simulink model "Beleuchtungs_Box17b"  (R2017b)
settings: Solver=FixedStepAuto  StartTime=0.0  StopTime=10.0  RelTol=1e-3
PreLoadFcn:
  | waijung.modelPreload; % Required for working with Waijung Blockset. Do not remove.
undefined symbols (not defined in the file): HSEOSC, Link, LQFP176, ST, STM32F417IG
libraries: simulink x18, canmsglib x10, stm32f4_canbus_lib x2, stm32f4_io_lib x1, stm32f4_device_config_lib x1, hdlsllib x1
CloseFcn:
  | waijung.modelClose; % Required for working with Waijung Blockset. Do not remove.
settings Model: Creator=labadmin  LastModifiedBy=MichaelRogalski
settings OptimizationCC: DefaultParameterBehavior=Inlined  PassReuseOutputArgsAs=Individual arguments
settings DebuggingCC: ParameterTunabilityLossMsg=error
settings HardwareCC: ProdBitPerPointer=32  ProdBitPerSizeT=32  ProdBitPerPtrDiffT=32  ProdLargestAtomicFloat=None  ProdIntDivRoundTo=Undefined  ProdWordSize=32  ProdHWDeviceType=ARM Compatible->Cortex - M4  TargetEndianess=LittleEndian  TargetHWDeviceType=ARM Compatible->Cortex - M4
settings SFSimCC: MATLABDynamicMemAlloc=off
settings RTWCC: Description=STM32F4 Target  SystemTargetFile=stm32f4.tlc  GenerateMakefile=off  TemplateMakefile=ert_default_tmf  GenerateReport=on  IncludeHyperlinkInReport=on  LaunchReport=on  GenerateTraceInfo=on  GenerateTraceReport=on  GenerateTraceReportSl=on  GenerateTraceReportSf=on  GenerateTraceReportEml=on
settings CodeAppCC: ForceParamTrailComments=on  IgnoreCustomStorageClasses=off  OperatorAnnotations=on  SimulinkDataObjDesc=on  SFDataObjDesc=on  InsertBlockDesc=on
settings STFCustomTargetCC: TargetLangStandard=C99 (ISO)  MultiwordLength=256  ModelReferenceCompliant=off  CombineOutputUpdateFcns=on  ERTCustomFileBanners=on  SupportContinuousTime=off  SupportNonInlinedSFcns=off  RemoveResetFunc=on  MATLABClassNameForMDSCustomization=Simulink.SoftwareTarget.ERTCustomization  GRTInterface=off  SystemTargetFile=stm32f4.tlc
settings ERTTargetCC: TargetLangStandard=C99 (ISO)  ModelReferenceCompliant=off  ParMdlRefBuildCompliant=off  CompOptLevelCompliant=off  ConcurrentExecutionCompliant=off  ModelStepFunctionPrototypeControlCompliant=off  CPPClassGenCompliant=off  UseToolchainInfoCompliant=off  InlinedParameterPlacement=NonHierarchical  ERTSrcFileBannerTemplate=stm32f4_code_template.cgt  ERTHdrFileBannerTemplate=stm32f4_code_template.cgt  ERTDataSrcFileTemplate=stm32f4_code_template.cgt  ERTDataHdrFileTemplate=stm32f4_code_template.cgt  ERTCustomFileTemplate=stm32f4_file_process.tlc

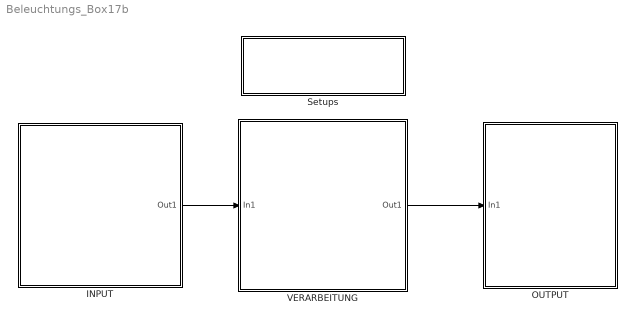
== system Beleuchtungs_Box17b ==
  INPUT : Subsystem
  OUTPUT : Subsystem
  Setups : Subsystem
  VERARBEITUNG : Subsystem
  wires:
  INPUT/1(Out1) -> VERARBEITUNG/1(In1)
  VERARBEITUNG/1(Out1) -> OUTPUT/1(In1)

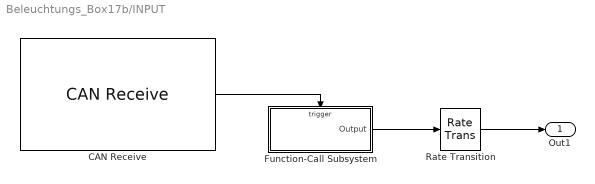
== system Beleuchtungs_Box17b/INPUT ==
  CAN Receive : stm32f4_canbus_lib/CAN Receive  conf=Rx  canmodule=1  idtype=Standard  filtertype=Mask  id=0  idmask=0  enableisr=on  usedlc=off  datatype=single  data0type=uint32  data1type=uint32  data2type=Not used  data3type=Not used  data4type=Not used  data5type=Not used  data6type=Not used  data7type=Not used  buffersize=8  sampletime=-1  sampletimestr=-1  blockid=INPUTCANReceive  inputarray=[]  inputlabelarray={}  outputarray=[7]  outputlabelarray={'Call ISR' }  compat=0  confstr=[]
      settings: SourceProductName=Waijung Blockset
  Function-Call Subsystem : Subsystem  TreatAsAtomicUnit=on
  Rate Transition : RateTransition
  Out1 : Outport  VectorParamsAs1DForOutWhenUnconnected=off
  wires:
  CAN Receive/1 -> Function-Call Subsystem/Trigger
  Function-Call Subsystem/1(Output) -> Rate Transition/1
  Rate Transition/1 -> Out1/1

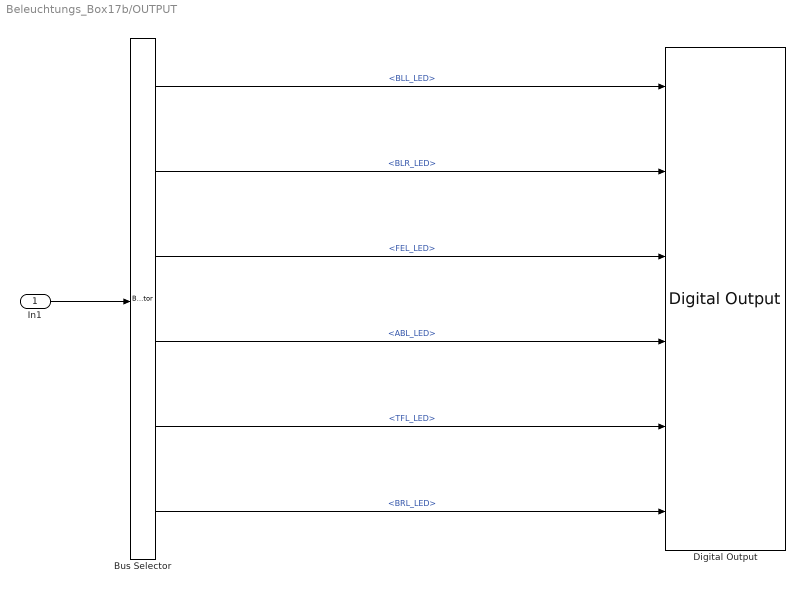
== system Beleuchtungs_Box17b/OUTPUT ==
  In1 : Inport
  Bus Selector : BusSelector  OutputSignals=BLL_LED,BLR_LED,FEL_LED,ABL_LED,TFL_LED,BRL_LED
  Digital Output : stm32f4_io_lib/Digital Output  use_bitband=on  port=C  speed=100  porttype=Push Pull  porttypestr=PP  use_pin0=on  use_pin1=on  use_pin2=on  use_pin3=on  use_pin4=on  use_pin5=on  use_pin6=off  use_pin7=off  use_pin8=off  use_pin9=off  use_pin10=off  use_pin11=off  use_pin12=off  use_pin13=off  use_pin14=off  use_pin15=off  pinstr=GPIO_Pin_0 | GPIO_Pin_1 | GPIO_Pin_2 | GPIO_Pin_3 | GPIO_Pin_4 | GPIO_Pin_5  usedpinarray="[1  1  1  1  1  1  0  0  0  0  0  0  0  0  0  0]"  bitbandingstr=|  sampletime=-1  sampletimestr=-1  blockid=OUTPUTDigitalOutput  enablecustomportlabel=off  globalinit=off  cinputportlabel=In1, In2  coutputportlabel=0
      | #define OUTPUTDigitalOutput_C0 Peripheral_BB(GPIOC->ODR, 0)  /* Output pin */
      | #define OUTPUTDigitalOutput_C1 Peripheral_BB(GPIOC->ODR, 1)  /* Output pin */
      | #define OUTPUTDigitalOutput_C2 Peripheral_BB(GPIOC->ODR, 2)  /* Output pin */
      | #define OUTPUTDigitalOutput_C3 Peripheral_BB(GPIOC->ODR, 3)  /* Output pin */
      | #define OUTPUTDigitalOutput_C4 Peripheral_BB(GPIOC->ODR, 4)  /* Output pin */
      | #define OUTPUTDigitalOutput_C5 Peripheral_BB(GPIOC->ODR, 5)  /* Output pin */
      settings: SourceProductName=Waijung Blockset
  wires:
  In1/1 -> Bus Selector/1
  Bus Selector/1 -> Digital Output/1  "<BLL_LED>"
  Bus Selector/2 -> Digital Output/2  "<BLR_LED>"
  Bus Selector/3 -> Digital Output/3  "<FEL_LED>"
  Bus Selector/4 -> Digital Output/4  "<ABL_LED>"
  Bus Selector/5 -> Digital Output/5  "<TFL_LED>"
  Bus Selector/6 -> Digital Output/6  "<BRL_LED>"

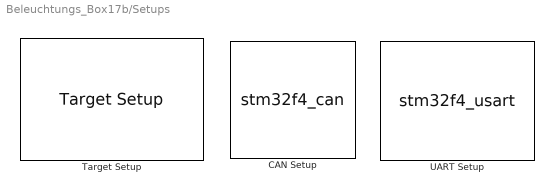
== system Beleuchtungs_Box17b/Setups ==
  CAN Setup : S-Function  FunctionName=stm32f4_can  Parameters=conf,canmodule,0,inputarray,outputarray,'','',confstr,sampletime,sampletimestr,blockid  SFunctionDeploymentMode=off  EnableBusSupport=off  mask(stm32f4_can){conf=Setup, canmodule=1, advance=off, bitrate_select=500000, sjw=1tq, bs1=14tq, bs2=6tq, timingconf=Prescaler, brp=4, bitrate=500000, tq=9.5238e-08, autoretransmission=Disable, remaptxpin=A12, remaprxpin=A11, sampletime=-1, sampletimestr=-1, blockid=SetupsCANSetup, inputarray=[], inputlabelarray={}, outputarray=[], outputlabelarray={}, compat=0, confstr=[], presc=4, txportstr=A, txpinstr=12, rxportstr=A, rxpinstr=11, lastmodule=1}
      mask prompts: conf "Configuration"; canmodule "CAN Module"; advance "Advance configuration"; bitrate_select "Baud rate (bps)"; sjw "Resync Jump Width (SJW)"; bs1 "Bit segment 1 (BS1) + PROP_SEG"; bs2 "Bit segment 2 (BS2)"; timingconf "Adjust"; brp "Baud rate prescaler (BRP)"; bitrate "Baud rate (bps)"; tq "Time Quantum (Second), tq"; autoretransmission "Auto Re-transmission"; remaptxpin "CAN Tx pin"; remaprxpin "CAN Rx pin"; sampletime "Sample time (sec)"; sampletimestr "Compiled sample time (sec) in string"; inputarray "Input port"; inputlabelarray "Input port label"; outputarray "Output port"; outputlabelarray "Output port label"; compat "Compatibility (Reserved for future use)"; confstr "Configuration String"; presc "Prescale"; txportstr "Tx port string"; txpinstr "Tx pin string"; rxportstr "Rx port string"; rxpinstr "Rx pin string"; lastmodule "Last module selected"
      mask help:
      | This block setups CAN Module.
      |
      | Auto Re-transmission,
      |  - Enable: The CAN hardware will automatically retransmit the message until it has been
      | successfully transmitted according to the CAN standard.
      |  - Disable: A message will be transmitted only once, independently of the transmission result
      | (successful, error or arbitration lost).
      mask init:
      | stm32f4_can_callback('init');
      mask Help: web(fullfile(waijungdocroot,'stm32f4_can_setup.htm'), '-browser')
      mask TypeOptions conf: Setup
      mask TypeOptions canmodule: 1 | 2
      mask Callback canmodule: stm32f4_can_callback('canmodule');
      mask Callback advance: stm32f4_can_callback('advance');
      mask TypeOptions bitrate_select: 125000 | 250000 | 500000 | 1000000
      mask Callback bitrate_select: stm32f4_can_callback('bitrate_select');
      mask TypeOptions sjw: 1tq | 2tq | 3tq | 4tq
      mask TypeOptions bs1: 1tq | 2tq | 3tq | 4tq | 5tq | 6tq | 7tq | 8tq | 9tq | 10tq | 11tq | 12tq | 13tq | 14tq | 15tq | 16tq
      mask Callback bs1: stm32f4_can_callback('timingconf');
      mask TypeOptions bs2: 1tq | 2tq | 3tq | 4tq | 5tq | 6tq | 7tq | 8tq
      mask Callback bs2: stm32f4_can_callback('timingconf');
      mask TypeOptions timingconf: Prescaler | Baudrate
      mask Callback timingconf: stm32f4_can_callback('timingconf');
      mask Callback brp: stm32f4_can_callback('timingconf');
      mask Callback bitrate: stm32f4_can_callback('timingconf');
      mask TypeOptions autoretransmission: Enable | Disable
      mask TypeOptions remaptxpin: Not used | A12 | B9 | D1 | H13
      mask Callback remaptxpin: stm32f4_can_callback('remaptxpin');
      mask TypeOptions remaprxpin: Not used | A11 | B8 | D0 | I9
      mask Callback remaprxpin: stm32f4_can_callback('remaprxpin');
      mask Callback sampletime: stm32f4_can_callback('sampletime');
      mask Callback sampletimestr: stm32f4_can_callback('sampletimestr');
      mask Callback blockid: stm32f4_can_callback('blockid');
      mask Display: text(0.5, 0.5, 'CAN1_Setup\nSpeed (bps): 500000\nTx/Rx pin: A12/A11','ver','middle','hor','center');
  Target Setup : stm32f4_device_config_lib/Target Setup  Priority=100  compiler=GNU ARM  previous_compiler=GNU ARM  mcu=STM32F417IG (LQFP176)  mcustr=STM32F417IG  clockconfig=HSEOSC-8MHz  system_stm32f4xx_c_path=D:\Downloads\waijung17_03a\targets\stm32f4_target\stm32f4\utils\system_stm32f4xx_default\STM32F40_41xxx\hseosc8mhz  showmemoryconfiguration=off  stacksize=0x2000  heapsize=0x2000  enableautocompiledownload=on  fullchiperase=off  programmerinterface=ST-Link  editctrlstr=on  compilercontrolstr=$(patsubst %, -I%, .) -mcpu=cortex-m4 -mthumb -mthumb-interwork -mfloat-abi=hard -mfpu=fpv4-sp-d16 -ffast-math -Wall -Wextra -Ofast  assemblercontrolstr=$(patsubst %, -I%, .) -mcpu=cortex-m4 -mthumb -mthumb-interwork -mfloat-abi=hard -mfpu=fpv4-sp-d16 -ffast-math -Wall -Wextra -Ofast -Wa,-amhls=$(<:.s=.lst) -D__STACK_SIZE=$(STACK_SIZE) -D__HEAP_SIZE=$(HEAP_SIZE)  linkercontrolstr=-T$(LD_SCRIPT) -g -Wl,-Map=$(MAP),--cref,--no-warn-mismatch -mcpu=cortex-m4 -mthumb -mthumb-interwork -mfloat-abi=hard -mfpu=fpv4-sp-d16 -specs=nosys.specs  runafterdownload=on  execprofile=None  profileruart=3  profilerbaud=500000  profilertxpin=D8  profilerinitstr=0.01,168000000,1680000,500000,0  manualsetsampletime=off  sampletime=0.01  blockid=SetupsTargetSetup  systickreloadvalue=1680000  hseval=8000000  lastprofileruart=3  hclk=168000000  flashorigin=0x8000000  flashlength=1024k  ramorigin=0x20000000  ramlength=128k  useextram=off
      settings: SourceProductName=Waijung Blockset
  UART Setup : S-Function  Priority=1  FunctionName=stm32f4_usart  Parameters=configuration,uartmodule,transfer,baudrate,inputtype,outputtype,confstr,binheaderarray,binterminatorarray,asciiheader,asciiterminator,bindatalength,packetmode,varname,sampletime,sampletimestr,blockid  SFunctionDeploymentMode=off  EnableBusSupport=off  mask(stm32f4_usart){configuration=Setup, uartmodule=2, baudrate=115200, databits=8, parity=No, stopbit=1, remaptxpin=A2, remaprxpin=A3, flowcontrol=None, remapctspin=Not used, remaprtspin=Not used, advanceoptions=off, rxbuffersize=512, txbuffersize=512, transfer=Blocking, packetmode=Ascii, binheader='7E 7E', binterminator='03 03', porttype_double=1, porttype_single=0, porttype_int8=1, porttype_uint8=0, porttype_int16=0, porttype_uint16=0, porttype_int32=0, porttype_uint32=0, asciiformat='%d,%f', rx_asciiterminator=CRLF (0x0D 0x0A - "\r\n"), tx_asciiterminator=CR (0x0D - "\r"), storagename=<empty>, varname=, inputtype=[0], outputtype=[0], binheaderarray=[0], binterminatorarray=[0], bindatalength=0, asciiheader='', asciiterminator=[0], sampletime=-1, sampletimestr=-1, blockid=SetupsUARTSetup, confstr=[ "dummy", "1", "A", "2", "1", "A", "3", "0", "*", "*", "0", "*", "*", "1", "4", "6", "1", "4", "5", "512", "512", "1", "2", "115200", "8", "No", "1", "None", "USART2"], lastmodule=2}
      mask prompts: uartmodule "UART Module"; baudrate "Baud rate (bps)"; databits "Data bits"; stopbit "Stop bit"; remaptxpin "Tx Pin"; remaprxpin "Rx Pin"; flowcontrol "Hardware flow control"; remapctspin "HW Flow control, CTS Pin"; remaprtspin "HW Flow control, RTS Pin"; advanceoptions "Advance options"; rxbuffersize "Rx buffer size (bytes)"; txbuffersize "Tx buffer size (bytes)"; packetmode "Packet mode"; binheader "Binary header (example: '7E 7E')"; binterminator "Binary terminator (example: '03 03')"; porttype_double "Number of data port, type DOUBLE"; porttype_single "Number of data port, type SINGLE"; porttype_int8 "Number of data port, type INT8"; porttype_uint8 "Number of data port, type UINT8"; porttype_int16 "Number of data port, type INT16"; porttype_uint16 "Number of data port, type UINT16"; porttype_int32 "Number of data port, type INT32"; porttype_uint32 "Number of data port, type UINT32"; asciiformat "Ascii format"; rx_asciiterminator "End of packet"; tx_asciiterminator "End of packet"; storagename "Buffer"; varname "Var name"; inputtype "Input data type"; outputtype "Output data type"; binheaderarray "Binary header"; binterminatorarray "Binary terminator"; bindatalength "Binary data length"; asciiheader "Ascii header (printf format)"; asciiterminator "Ascii terminator"; sampletime "Sample time (sec)"; sampletimestr "Compiled sample time (sec) in string"; confstr "Configuration string"; lastmodule "Last module selected"
      mask help:
      | Default STM32F4DISCOVERY + aMG F4 Connect 2 + aMG USB Converter N2 settings use
      |
      | USART3, Tx D8, Rx D9 and USB Serial Converter A.
      mask init:
      | stm32f4_usart_callback('init');
      mask Help: web(fullfile(waijungdocroot,'stm32f4_usart_setup.htm'), '-browser')
      mask TypeOptions configuration: Setup | Tx | Rx
      mask Callback configuration: stm32f4_usart_callback('configuration');
      mask TypeOptions uartmodule: 1 | 2 | 3 | 4 | 5 | 6
      mask Callback uartmodule: stm32f4_usart_callback('uartmodule');
      mask Callback baudrate: stm32f4_usart_callback('baudrate');
      mask TypeOptions databits: 8
      mask TypeOptions parity: No | Odd | Even
      mask TypeOptions stopbit: 0.5 | 1 | 1.5 | 2
      mask TypeOptions remaptxpin: Not used | A2 | D5
      mask TypeOptions remaprxpin: Not used | A3 | D6
      mask TypeOptions flowcontrol: None | RTS | CTS | RTS/CTS
      mask Callback flowcontrol: stm32f4_usart_callback('flowcontrol');
      mask TypeOptions remapctspin: Not used | A0 | D3
      mask TypeOptions remaprtspin: Not used | A1 | D4
      mask Callback advanceoptions: stm32f4_usart_callback('advanceoptions');
      mask TypeOptions rxbuffersize: 16 | 32 | 64 | 128 | 256 | 512 | 1024 | 2048
      mask TypeOptions txbuffersize: 16 | 32 | 64 | 128 | 256 | 512 | 1024 | 2048
      mask TypeOptions transfer: Blocking | Non-Blocking
      mask Callback transfer: stm32f4_usart_callback('transfer');
      mask TypeOptions packetmode: Ascii | Binary | String Buffer
      mask Callback packetmode: stm32f4_usart_callback('packetmode');
      mask Callback binheader: stm32f4_usart_callback('binheader');
      mask Callback binterminator: stm32f4_usart_callback('binterminator');
      mask Callback porttype_double: stm32f4_usart_callback('porttype');
      mask Callback porttype_single: stm32f4_usart_callback('porttype');
      mask Callback porttype_int8: stm32f4_usart_callback('porttype');
      mask Callback porttype_uint8: stm32f4_usart_callback('porttype');
      mask Callback porttype_int16: stm32f4_usart_callback('porttype');
      mask Callback porttype_uint16: stm32f4_usart_callback('porttype');
      mask Callback porttype_int32: stm32f4_usart_callback('porttype');
      mask Callback porttype_uint32: stm32f4_usart_callback('porttype');
      mask Callback asciiformat: stm32f4_usart_callback('asciiformat');
      mask TypeOptions rx_asciiterminator: CR (0x0D - "\r") | LF (0x0A - "\n") | CRLF (0x0D 0x0A - "\r\n")
      mask Callback rx_asciiterminator: stm32f4_usart_callback('rx_asciiterminator');
      mask TypeOptions tx_asciiterminator: CR (0x0D - "\r") | LF (0x0A - "\n") | CRLF (0x0D 0x0A - "\r\n") | None
      mask Callback tx_asciiterminator: stm32f4_usart_callback('tx_asciiterminator');
      mask TypeOptions storagename: <empty>
      mask Callback storagename: stm32f4_usart_callback('storagename');
      mask Callback varname: stm32f4_usart_callback('varname');
      mask Callback sampletime: stm32f4_usart_callback('sampletime');
      mask Callback sampletimestr: stm32f4_usart_callback('sampletimestr');
      mask Callback blockid: stm32f4_usart_callback('blockid');
      mask Display: text(0.5, 0.5, 'Module: USART2_Setup\nBaud (Bps): 115200\nDMA Buffer: 512/512\nTx/Rx Pin: A2/A3','ver','middle','hor','center');

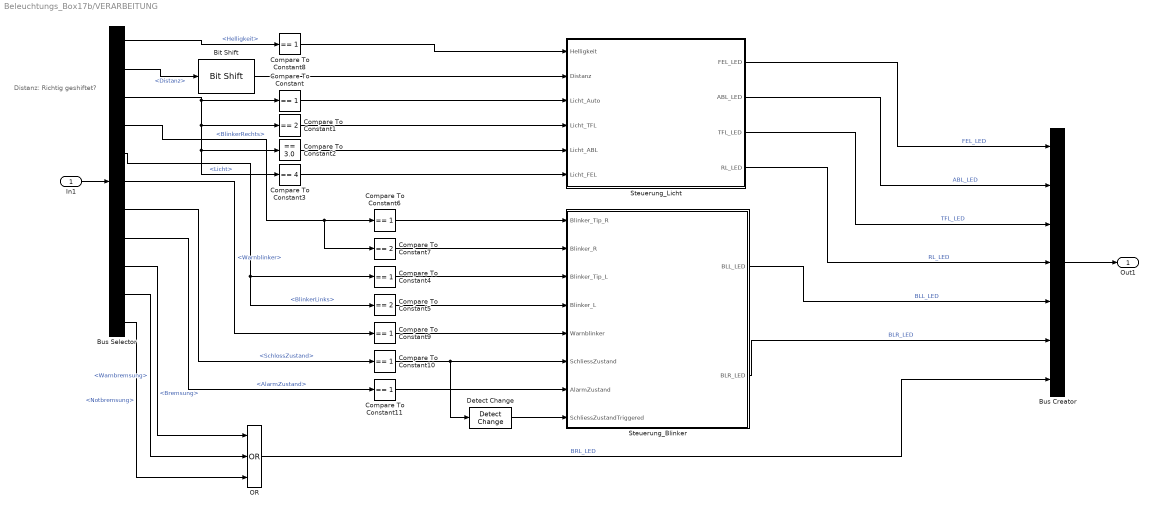
== system Beleuchtungs_Box17b/VERARBEITUNG ==
  note: Distanz: Richtig geshiftet?
  In1 : Inport
  Bit Shift : hdlsllib/Logic and Bit Operations/Bit Shift  mode=Shift Right Logical  N=1
      settings: SourceProductName=Simulink
  Bus Creator : BusCreator  Inputs=7
  Bus Selector : BusSelector  OutputSignals=Helligkeit,Distanz,Licht,BlinkerRechts,BlinkerLinks,Warnblinker,SchlossZustand,AlarmZustand,Bremsung,Warnbremsung,Notbremsung
  Compare To Constant{,4,6,8..11} (7 alike) : simulink/Logic and Bit Operations/Compare To Constant  relop===  const=1  OutDataTypeStr=boolean
  Compare To Constant1 : simulink/Logic and Bit Operations/Compare To Constant  relop===  const=2  OutDataTypeStr=boolean
  Compare To Constant2 : simulink/Logic and Bit Operations/Compare To Constant  relop===  const=3.0  OutDataTypeStr=boolean
  Compare To Constant3 : simulink/Logic and Bit Operations/Compare To Constant  relop===  const=4  OutDataTypeStr=boolean
  Compare To Constant5 : simulink/Logic and Bit Operations/Compare To Constant  relop===  const=2  OutDataTypeStr=boolean
  Compare To Constant7 : simulink/Logic and Bit Operations/Compare To Constant  relop===  const=2  OutDataTypeStr=boolean
  Detect Change : simulink/Logic and Bit Operations/Detect Change  vinit=0  OutDataTypeStr=boolean
  OR : Logic  Operator=OR  Inputs=3  IconShape=distinctive  AllPortsSameDT=off  OutDataTypeStr=boolean
  Steuerung_Blinker : Stateflow chart  TreatAsAtomicUnit=on
  Steuerung_Licht : Stateflow chart  TreatAsAtomicUnit=on
  Out1 : Outport  VectorParamsAs1DForOutWhenUnconnected=off
  wires:
  Bus Creator/1 -> Out1/1
  In1/1 -> Bus Selector/1
  Steuerung_Licht/3(TFL_LED) -> Bus Creator/3  "TFL_LED"
  Steuerung_Licht/4(RL_LED) -> Bus Creator/4  "RL_LED"
  Steuerung_Licht/1(FEL_LED) -> Bus Creator/1  "FEL_LED"
  Steuerung_Licht/2(ABL_LED) -> Bus Creator/2  "ABL_LED"
  Steuerung_Blinker/1(BLL_LED) -> Bus Creator/5  "BLL_LED"
  Steuerung_Blinker/2(BLR_LED) -> Bus Creator/6  "BLR_LED"
  Compare To Constant3/1 -> Steuerung_Licht/6(Licht_FEL)
  Compare To Constant2/1 -> Steuerung_Licht/5(Licht_ABL)
  Compare To Constant1/1 -> Steuerung_Licht/4(Licht_TFL)
  Compare To Constant/1 -> Steuerung_Licht/3(Licht_Auto)
  Bus Selector/3 -> Compare To Constant3/1, Compare To Constant2/1, Compare To Constant1/1, Compare To Constant/1  "<Licht>"
  Bus Selector/1 -> Compare To Constant8/1  "<Helligkeit>"
  Bus Selector/4 -> Compare To Constant6/1, Compare To Constant7/1  "<BlinkerRechts>"
  Bus Selector/5 -> Compare To Constant4/1, Compare To Constant5/1  "<BlinkerLinks>"
  Compare To Constant4/1 -> Steuerung_Blinker/3(Blinker_Tip_L)
  Compare To Constant5/1 -> Steuerung_Blinker/4(Blinker_L)
  Compare To Constant6/1 -> Steuerung_Blinker/1(Blinker_Tip_R)
  Compare To Constant7/1 -> Steuerung_Blinker/2(Blinker_R)
  Bus Selector/6 -> Compare To Constant9/1  "<Warnblinker>"
  Compare To Constant9/1 -> Steuerung_Blinker/5(Warnblinker)
  Bus Selector/7 -> Compare To Constant10/1  "<SchlossZustand>"
  Bus Selector/8 -> Compare To Constant11/1  "<AlarmZustand>"
  Compare To Constant10/1 -> Detect Change/1, Steuerung_Blinker/6(SchliessZustand)
  Compare To Constant11/1 -> Steuerung_Blinker/7(AlarmZustand)
  Detect Change/1 -> Steuerung_Blinker/8(SchliessZustandTriggered)
  Compare To Constant8/1 -> Steuerung_Licht/1(Helligkeit)
  Bus Selector/2 -> Bit Shift/1  "<Distanz>"
  Bit Shift/1 -> Steuerung_Licht/2(Distanz)
  Bus Selector/9 -> OR/1  "<Bremsung>"
  Bus Selector/10 -> OR/2  "<Warnbremsung>"
  Bus Selector/11 -> OR/3  "<Notbremsung>"
  OR/1 -> Bus Creator/7  "BRL_LED"

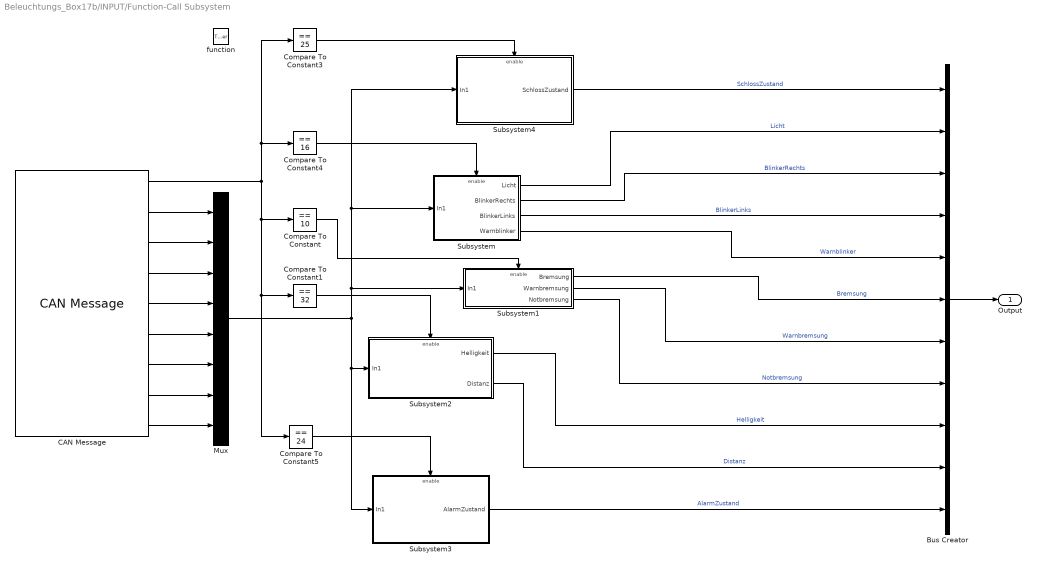
== system Beleuchtungs_Box17b/INPUT/Function-Call Subsystem ==
  function : TriggerPort  TriggerType=function-call  VariantControl=Variant
  Bus Creator : BusCreator  Inputs=11
  CAN Message : stm32f4_canbus_lib/CAN Message  conf=Msg  canmodule=1  usedlc=off  datatype=double  data0type=uint8  data1type=uint8  data2type=uint8  data3type=uint8  data4type=uint8  data5type=uint8  data6type=uint8  data7type=uint8  sampletime=-1  sampletimestr=-1  blockid=INPUTFunctionCallSubsystemCANMessage  inputarray=[]  inputlabelarray={}  outputarray=[ 7, 3, 3, 3, 3, 3, 3, 3, 3]  outputlabelarray={'ID', 'D0 (uint8)', 'D1 (uint8)', 'D2 (uint8)', 'D3 (uint8)', 'D4 (uint8)', 'D5 (uint8)', 'D6 (uint8)', 'D7 (uint8)' }  compat=0  confstr=[]
      settings: SourceProductName=Waijung Blockset
  Compare To Constant : simulink/Logic and Bit Operations/Compare To Constant  relop===  const=10  OutDataTypeStr=boolean
  Compare To Constant1 : simulink/Logic and Bit Operations/Compare To Constant  relop===  const=32  OutDataTypeStr=boolean
  Compare To Constant3 : simulink/Logic and Bit Operations/Compare To Constant  relop===  const=25  OutDataTypeStr=boolean
  Compare To Constant4 : simulink/Logic and Bit Operations/Compare To Constant  relop===  const=16  OutDataTypeStr=boolean
  Compare To Constant5 : simulink/Logic and Bit Operations/Compare To Constant  relop===  const=24  OutDataTypeStr=boolean
  Mux : Mux  Inputs=8
  Subsystem : Subsystem
  Subsystem1 : Subsystem
  Subsystem2 : Subsystem
  Subsystem3 : Subsystem
  Subsystem4 : Subsystem
  Output : Outport  VectorParamsAs1DForOutWhenUnconnected=off
  wires:
  CAN Message/1 -> Compare To Constant5/1, Compare To Constant1/1, Compare To Constant/1, Compare To Constant4/1, Compare To Constant3/1
  CAN Message/3 -> Mux/2
  CAN Message/2 -> Mux/1
  CAN Message/4 -> Mux/3
  CAN Message/5 -> Mux/4
  CAN Message/6 -> Mux/5
  CAN Message/7 -> Mux/6
  CAN Message/8 -> Mux/7
  CAN Message/9 -> Mux/8
  Bus Creator/1 -> Output/1
  Compare To Constant4/1 -> Subsystem/Enable
  Compare To Constant/1 -> Subsystem1/Enable
  Compare To Constant1/1 -> Subsystem2/Enable
  Subsystem4/1(SchlossZustand) -> Bus Creator/1  "SchlossZustand"
  Subsystem/1(Licht) -> Bus Creator/2  "Licht"
  Subsystem/2(BlinkerRechts) -> Bus Creator/3  "BlinkerRechts"
  Subsystem/3(BlinkerLinks) -> Bus Creator/4  "BlinkerLinks"
  Subsystem/4(Warnblinker) -> Bus Creator/5  "Warnblinker"
  Subsystem1/1(Bremsung) -> Bus Creator/6  "Bremsung"
  Subsystem1/2(Warnbremsung) -> Bus Creator/7  "Warnbremsung"
  Subsystem1/3(Notbremsung) -> Bus Creator/8  "Notbremsung"
  Subsystem2/1(Helligkeit) -> Bus Creator/9  "Helligkeit"
  Subsystem2/2(Distanz) -> Bus Creator/10  "Distanz"
  Subsystem3/1(AlarmZustand) -> Bus Creator/11  "AlarmZustand"
  Compare To Constant5/1 -> Subsystem3/Enable
  Compare To Constant3/1 -> Subsystem4/Enable
  Mux/1 -> Subsystem3/1(In1), Subsystem2/1(In1), Subsystem4/1(In1), Subsystem/1(In1), Subsystem1/1(In1)

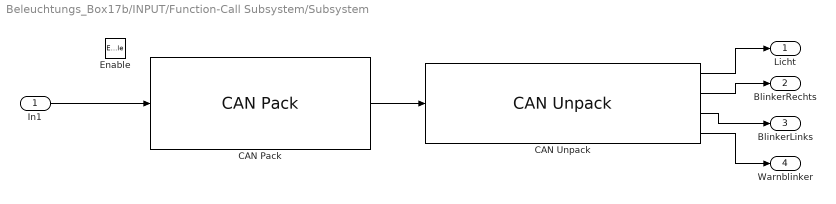
== system Beleuchtungs_Box17b/INPUT/Function-Call Subsystem/Subsystem ==
  In1 : Inport
  Enable : EnablePort
  CAN Pack : canmsglib/CAN Pack  MsgList=(none)  MsgName=CAN_Data_Cockpit1  MsgIDType=Standard (11-bit identifier)  MsgIdentifier=16  MsgLength=1  Remote=off  ApplyMinMax=off  BusOutput=off  NSignals=0  StartBits=0  SignalSizes=0  ByteOrders=0  DataTypes=0  MultiplexTypes=0  MultiplexValues=0  Factors=0  Offsets=0  Minimums=0  Maximums=0
      settings: SourceProductName=Simulink Real-Time  SourceProductBaseCode=XP  DataFormat=raw data
  CAN Unpack : canmsglib/CAN Unpack  MsgList=(none)  MsgName=CAN_Data_Cockpit1  MsgIDType=Standard (11-bit identifier)  MsgIdentifier=16  MsgLength=1  SignalInfo=Licht$0$3$1$2$1$0$1$0$-Inf$Inf$#BlinkerRechts$3$2$1$2$1$0$1$0$-Inf$Inf$#BlinkerLinks$5$2$1$2$1$0$1$0$-Inf$Inf$#Warnblinker$7$1$1$2$1$0$1$0$-Inf$Inf$#  IDPort=off  TimestampPort=off  ErrorPort=off  RemotePort=off  LengthPort=off  StatusPort=off  ApplyMinMax=off  NSignals=4  StartBits=str2num('[int32(0);int32(3);int32(5);int32(7)]')  SignalSizes=str2num('[int32(3);int32(2);int32(2);int32(1)]')  ByteOrders=str2num('[int32(1);int32(1);int32(1);int32(1)]')  DataTypes=str2num('[int32(2);int32(2);int32(2);int32(2)]')  MultiplexTypes=str2num('[int32(1);int32(1);int32(1);int32(1)]')  MultiplexValues=str2num('[double(0);double(0);double(0);double(0)]')  Factors=str2num('[double(1);double(1);double(1);double(1)]')  Offsets=str2num('[double(0);double(0);double(0);double(0)]')  Minimums=str2num('[double(-Inf);double(-Inf);double(-Inf);double(-Inf)]')  Maximums=str2num('[double(Inf);double(Inf);double(Inf);double(Inf)]')
      settings: SourceProductName=Simulink Real-Time  SourceProductBaseCode=XP
  Licht : Outport  VectorParamsAs1DForOutWhenUnconnected=off
  BlinkerRechts : Outport  Port=2  VectorParamsAs1DForOutWhenUnconnected=off
  BlinkerLinks : Outport  Port=3  VectorParamsAs1DForOutWhenUnconnected=off
  Warnblinker : Outport  Port=4  VectorParamsAs1DForOutWhenUnconnected=off
  wires:
  CAN Pack/1 -> CAN Unpack/1
  In1/1 -> CAN Pack/1
  CAN Unpack/4 -> Warnblinker/1
  CAN Unpack/3 -> BlinkerLinks/1
  CAN Unpack/2 -> BlinkerRechts/1
  CAN Unpack/1 -> Licht/1

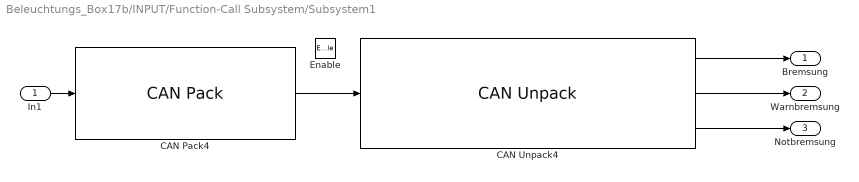
== system Beleuchtungs_Box17b/INPUT/Function-Call Subsystem/Subsystem1 ==
  In1 : Inport
  Enable : EnablePort
  CAN Pack4 : canmsglib/CAN Pack  MsgList=(none)  MsgName=CAN_Data_Bremse1  MsgIDType=Standard (11-bit identifier)  MsgIdentifier=10  MsgLength=1  Remote=off  ApplyMinMax=off  BusOutput=off  NSignals=0  StartBits=0  SignalSizes=0  ByteOrders=0  DataTypes=0  MultiplexTypes=0  MultiplexValues=0  Factors=0  Offsets=0  Minimums=0  Maximums=0
      settings: SourceProductName=Simulink Real-Time  SourceProductBaseCode=XP  DataFormat=raw data
  CAN Unpack4 : canmsglib/CAN Unpack  MsgList=(none)  MsgName=CAN_Data_Bremse1  MsgIDType=Standard (11-bit identifier)  MsgIdentifier=10  MsgLength=1  SignalInfo=Bremsung$0$1$1$2$1$0$1$0$-Inf$Inf$#WarnBremsung$1$1$1$2$1$0$1$0$-Inf$Inf$#NotBremsung$2$1$1$2$1$0$1$0$-Inf$Inf$#  IDPort=off  TimestampPort=off  ErrorPort=off  RemotePort=off  LengthPort=off  StatusPort=off  ApplyMinMax=off  NSignals=3  StartBits=str2num('[int32(0);int32(1);int32(2)]')  SignalSizes=str2num('[int32(1);int32(1);int32(1)]')  ByteOrders=str2num('[int32(1);int32(1);int32(1)]')  DataTypes=str2num('[int32(2);int32(2);int32(2)]')  MultiplexTypes=str2num('[int32(1);int32(1);int32(1)]')  MultiplexValues=str2num('[double(0);double(0);double(0)]')  Factors=str2num('[double(1);double(1);double(1)]')  Offsets=str2num('[double(0);double(0);double(0)]')  Minimums=str2num('[double(-Inf);double(-Inf);double(-Inf)]')  Maximums=str2num('[double(Inf);double(Inf);double(Inf)]')
      settings: SourceProductName=Simulink Real-Time  SourceProductBaseCode=XP
  Bremsung : Outport  VectorParamsAs1DForOutWhenUnconnected=off
  Warnbremsung : Outport  Port=2  VectorParamsAs1DForOutWhenUnconnected=off
  Notbremsung : Outport  Port=3  VectorParamsAs1DForOutWhenUnconnected=off
  wires:
  CAN Pack4/1 -> CAN Unpack4/1
  CAN Unpack4/2 -> Warnbremsung/1
  CAN Unpack4/1 -> Bremsung/1
  CAN Unpack4/3 -> Notbremsung/1
  In1/1 -> CAN Pack4/1

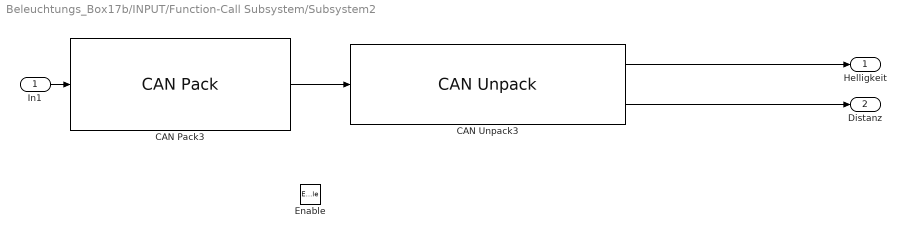
== system Beleuchtungs_Box17b/INPUT/Function-Call Subsystem/Subsystem2 ==
  In1 : Inport
  Enable : EnablePort
  CAN Pack3 : canmsglib/CAN Pack  MsgList=(none)  MsgName=CAN_Data_Sensor1  MsgIDType=Standard (11-bit identifier)  MsgIdentifier=32  MsgLength=2  Remote=off  ApplyMinMax=off  BusOutput=off  NSignals=0  StartBits=0  SignalSizes=0  ByteOrders=0  DataTypes=0  MultiplexTypes=0  MultiplexValues=0  Factors=0  Offsets=0  Minimums=0  Maximums=0
      settings: SourceProductName=Simulink Real-Time  SourceProductBaseCode=XP  DataFormat=raw data
  CAN Unpack3 : canmsglib/CAN Unpack  MsgList=(none)  MsgName=CAN_Data_Sensor1  MsgIDType=Standard (11-bit identifier)  MsgIdentifier=32  MsgLength=2  SignalInfo=Helligkeit$0$1$1$2$1$0$1$0$-Inf$Inf$#Distanz$1$9$1$2$1$0$1$0$-Inf$Inf$#  IDPort=off  TimestampPort=off  ErrorPort=off  RemotePort=off  LengthPort=off  StatusPort=off  ApplyMinMax=off  NSignals=2  StartBits=str2num('[int32(0);int32(1)]')  SignalSizes=str2num('[int32(1);int32(9)]')  ByteOrders=str2num('[int32(1);int32(1)]')  DataTypes=str2num('[int32(2);int32(2)]')  MultiplexTypes=str2num('[int32(1);int32(1)]')  MultiplexValues=str2num('[double(0);double(0)]')  Factors=str2num('[double(1);double(1)]')  Offsets=str2num('[double(0);double(0)]')  Minimums=str2num('[double(-Inf);double(-Inf)]')  Maximums=str2num('[double(Inf);double(Inf)]')
      settings: SourceProductName=Simulink Real-Time  SourceProductBaseCode=XP
  Helligkeit : Outport  VectorParamsAs1DForOutWhenUnconnected=off
  Distanz : Outport  Port=2  VectorParamsAs1DForOutWhenUnconnected=off
  wires:
  In1/1 -> CAN Pack3/1
  CAN Pack3/1 -> CAN Unpack3/1
  CAN Unpack3/1 -> Helligkeit/1
  CAN Unpack3/2 -> Distanz/1

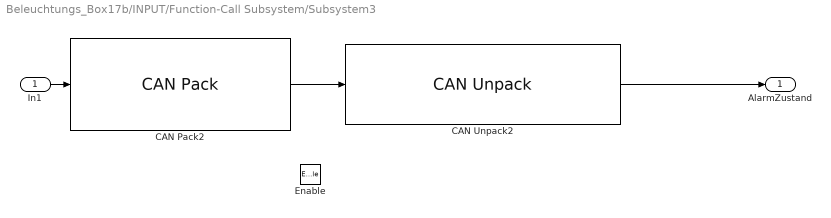
== system Beleuchtungs_Box17b/INPUT/Function-Call Subsystem/Subsystem3 ==
  In1 : Inport
  Enable : EnablePort
  CAN Pack2 : canmsglib/CAN Pack  MsgList=(none)  MsgName=CAN_Data_Alarm1  MsgIDType=Standard (11-bit identifier)  MsgIdentifier=24  MsgLength=1  Remote=off  ApplyMinMax=off  BusOutput=off  NSignals=0  StartBits=0  SignalSizes=0  ByteOrders=0  DataTypes=0  MultiplexTypes=0  MultiplexValues=0  Factors=0  Offsets=0  Minimums=0  Maximums=0
      settings: SourceProductName=Simulink Real-Time  SourceProductBaseCode=XP  DataFormat=raw data
  CAN Unpack2 : canmsglib/CAN Unpack  MsgList=(none)  MsgName=CAN_Data_Alarm1  MsgIDType=Standard (11-bit identifier)  MsgIdentifier=24  MsgLength=1  SignalInfo=AlarmZustand$0$1$1$2$1$0$1$0$-Inf$Inf$#  IDPort=off  TimestampPort=off  ErrorPort=off  RemotePort=off  LengthPort=off  StatusPort=off  ApplyMinMax=off  NSignals=1  StartBits=str2num('[int32(0)]')  SignalSizes=str2num('[int32(1)]')  ByteOrders=str2num('[int32(1)]')  DataTypes=str2num('[int32(2)]')  MultiplexTypes=str2num('[int32(1)]')  MultiplexValues=str2num('[double(0)]')  Factors=str2num('[double(1)]')  Offsets=str2num('[double(0)]')  Minimums=str2num('[double(-Inf)]')  Maximums=str2num('[double(Inf)]')
      settings: SourceProductName=Simulink Real-Time  SourceProductBaseCode=XP
  AlarmZustand : Outport  VectorParamsAs1DForOutWhenUnconnected=off
  wires:
  CAN Pack2/1 -> CAN Unpack2/1
  In1/1 -> CAN Pack2/1
  CAN Unpack2/1 -> AlarmZustand/1

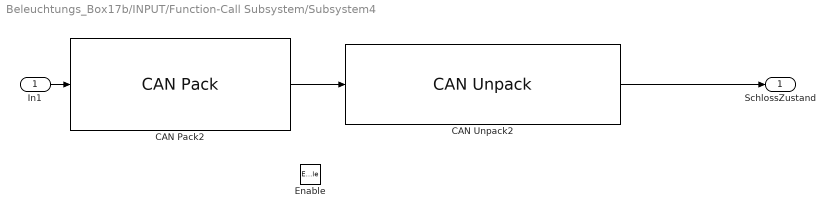
== system Beleuchtungs_Box17b/INPUT/Function-Call Subsystem/Subsystem4 ==
  In1 : Inport
  Enable : EnablePort
  CAN Pack2 : canmsglib/CAN Pack  MsgList=(none)  MsgName=CAN_Data_Schloss1  MsgIDType=Standard (11-bit identifier)  MsgIdentifier=25  MsgLength=1  Remote=off  ApplyMinMax=off  BusOutput=off  NSignals=0  StartBits=0  SignalSizes=0  ByteOrders=0  DataTypes=0  MultiplexTypes=0  MultiplexValues=0  Factors=0  Offsets=0  Minimums=0  Maximums=0
      settings: SourceProductName=Simulink Real-Time  SourceProductBaseCode=XP  DataFormat=raw data
  CAN Unpack2 : canmsglib/CAN Unpack  MsgList=(none)  MsgName=CAN_Data_Schloss1  MsgIDType=Standard (11-bit identifier)  MsgIdentifier=25  MsgLength=1  SignalInfo=SchlossZustand$0$1$1$2$1$0$1$0$-Inf$Inf$#  IDPort=off  TimestampPort=off  ErrorPort=off  RemotePort=off  LengthPort=off  StatusPort=off  ApplyMinMax=off  NSignals=1  StartBits=str2num('[int32(0)]')  SignalSizes=str2num('[int32(1)]')  ByteOrders=str2num('[int32(1)]')  DataTypes=str2num('[int32(2)]')  MultiplexTypes=str2num('[int32(1)]')  MultiplexValues=str2num('[double(0)]')  Factors=str2num('[double(1)]')  Offsets=str2num('[double(0)]')  Minimums=str2num('[double(-Inf)]')  Maximums=str2num('[double(Inf)]')
      settings: SourceProductName=Simulink Real-Time  SourceProductBaseCode=XP
  SchlossZustand : Outport  VectorParamsAs1DForOutWhenUnconnected=off
  wires:
  CAN Unpack2/1 -> SchlossZustand/1
  In1/1 -> CAN Pack2/1
  CAN Pack2/1 -> CAN Unpack2/1

== stateflow chart Beleuchtungs_Box17b/VERARBEITUNG/Steuerung_Licht ==
  state State_Licht_ABL
    entry:
    FEL_LED=false;
    ABL_LED=true;
    TFL_LED=false;
    RL_LED = true
  state State_Licht_Auto
    state Dunkel
      entry: RL_LED = true
      state Gegenverkehr_nein
        entry:
        FEL_LED=true;
        ABL_LED=false;
        TFL_LED=false;
      state Gegenverkehr_Ja
        entry:
        FEL_LED=false;
        ABL_LED=true;
        TFL_LED=false;
      Gegenverkehr_nein -> Gegenverkehr_Ja : [Distanz < 250]
      Gegenverkehr_Ja -> Gegenverkehr_nein : [Distanz > 250]
      (default) -> Gegenverkehr_Ja
    state Hell
      entry:
      FEL_LED = false;
      ABL_LED = false;
      TFL_LED = true;
      RL_LED = false
    (default) -> Hell
    Hell -> Dunkel : [Helligkeit == 1]
    Dunkel -> Hell : [Helligkeit == 0]
  state State_OFF
    entry:
    FEL_LED=false;
    ABL_LED=false;
    TFL_LED=false;
  state State_Licht_FEL
    entry:
    FEL_LED=true;
    ABL_LED=false;
    TFL_LED=false;
    RL_LED = true
  state State_Licht_TFL
    entry:
    FEL_LED=false;
    ABL_LED=false;
    TFL_LED=true;
    RL_LED = false
  State_Licht_ABL -> State_OFF : [Licht_ABL == 0]
  State_OFF -> State_Licht_ABL [order 1] : [Licht_ABL == 1]
  (default) -> State_OFF
  State_OFF -> State_Licht_FEL [order 2] : [Licht_FEL == 1]
  State_Licht_Auto -> State_OFF : [Licht_Auto == 0]
  State_OFF -> State_Licht_Auto [order 4] : [Licht_Auto==1]
  State_Licht_FEL -> State_OFF : [Licht_FEL==0]
  State_OFF -> State_Licht_TFL [order 3] : [Licht_TFL==1]
  State_Licht_TFL -> State_OFF : [Licht_TFL== 0]
  data: FEL_LED output boolean; Helligkeit input boolean; Distanz input uint16; ABL_LED output boolean; TFL_LED output boolean; Licht_Auto input boolean; Licht_TFL input boolean; Licht_ABL input boolean; Licht_FEL input boolean; RL_LED output boolean

== stateflow chart Beleuchtungs_Box17b/VERARBEITUNG/Steuerung_Blinker ==
  state State_Blinker_Bedienung
    state State_OFF
      en, du:
      Blinker_Aktiv = false
    state State_Blinken_Rechts
      en, du:
      Rechte_Seite_an = true
      Linke_Seite_an = false
      Blink_Frequenz =0.5
      Blinker_Aktiv = true
    state State_Blinken_Links
      en, du:
      Rechte_Seite_an = false
      Linke_Seite_an = true
      Blink_Frequenz =0.5
      Blinker_Aktiv = true
    state State_Warnblinken
      en, du:
      Rechte_Seite_an = true
      Linke_Seite_an = true
      Blink_Frequenz =0.5
      Blinker_Aktiv = true
    state State_Alarmblinken
      en, du:
      Rechte_Seite_an = true
      Linke_Seite_an = true
      Blink_Frequenz =0.25
      Blinker_Aktiv = true
    state State_Komfort_Links
      en, du:
      Rechte_Seite_an = false
      Linke_Seite_an = true
      Blink_Frequenz =0.5
      Blinker_Aktiv = true
      blink_count = 2
      flag = true
    state State_Komfort_Rechts
      en, du:
      Rechte_Seite_an = true
      Linke_Seite_an = false
      Blink_Frequenz =0.5
      Blinker_Aktiv = true
      blink_count = 2
      flag = false
    state State_Blinker_Oeffnen_Schliessen
      en, du: Rechte_Seite_an = true
      Linke_Seite_an = true
      Blink_Frequenz =0.5
      if SchliessZustand == true
      blink_count = 1
      end
      Blinker_Aktiv = true
    (junction 202) -> State_OFF [order 8]
    (junction 202) -> State_Blinken_Rechts [order 3] : [Blinker_R]
    (junction 202) -> State_Blinken_Links [order 4] : [Blinker_L]
    (default) -> (junction 202)
    State_Blinker_Bedienung -> (junction 202) [order 1]
    (junction 202) -> State_Warnblinken [order 1] : [Warnblinker]
    (junction 202) -> State_Alarmblinken [order 2] : [AlarmZustand]
    (junction 202) -> State_Komfort_Links [order 5] : [Blinker_Tip_L]
    (junction 202) -> State_Komfort_Rechts [order 6] : [Blinker_Tip_R]
    (junction 202) -> State_Blinker_Oeffnen_Schliessen [order 7] : [SchliessZustandTriggered]
  state State_Blinker_ON
    en, du:
    BLL_LED=Linke_Seite_an
    BLR_LED=Rechte_Seite_an
  state State_Blinker_OFF
    en, du:
    BLL_LED=false
    BLR_LED=false
    if flag == true
    BlinkerLinks = true
    end
    if flag == false
    BlinkerRechts = true
    end
  (default) -> State_Blinker_Bedienung : {Blinker_Aktiv =false, BlinkerLinks = false, BlinkerRechts = false, flag = false, blink_count = 0}
  State_Blinker_ON -> State_Blinker_Bedienung [order 1] : [(Warnblinker || Blinker_L || Blinker_R) && blink_count > 0]{blink_count = 0, BlinkerLinks = false, BlinkerRechts = false}
  State_Blinker_OFF -> State_Blinker_ON [order 2] : [blink_count > 0 && after(Blink_Frequenz, sec)]{blink_count = blink_count - 1}
  State_Blinker_Bedienung -> State_Blinker_ON [order 1] : [Blinker_Aktiv == true]
  State_Blinker_ON -> State_Blinker_OFF [order 2] : [ after(Blink_Frequenz,sec)]
  State_Blinker_OFF -> State_Blinker_Bedienung [order 3] : [after(Blink_Frequenz, sec)]{BlinkerLinks = false, BlinkerRechts = false}
  State_Blinker_OFF -> State_Blinker_Bedienung [order 1] : [(Warnblinker || Blinker_L || Blinker_R || (BlinkerLinks == true && Blinker_Tip_R) || (BlinkerRechts == true && Blinker_Tip_L) )  && blink_count > 0]{blink_count = 0, BlinkerLinks = false, BlinkerRechts = false}
  data: BLL_LED output boolean; BLR_LED output boolean; Blinker_Tip_R input; Blinker_R input; Blinker_Tip_L input; Blinker_L input; Warnblinker input boolean; SchliessZustand input boolean; AlarmZustand input boolean; Count local; OpeningCount local; ClosingCount local; Opening local; Closing local; blink_left local boolean; blink_right local boolean; blink_count local uint32; blink_delay local double; SchliessZustandTriggered input; Blink_Frequenz local double; Blinker_Aktiv local boolean; Rechte_Seite_an local boolean; Linke_Seite_an local boolean; Blinker_Stopp local; BlinkCounter local; BlinkerLinks local boolean; BlinkerRechts local boolean; flag local boolean
  events: SchliessZustandUpdated local FUNCTION_CALL_EVENT; AlarmZustandUpdated local FUNCTION_CALL_EVENT
